simulink model "simulink_scope"  (R2015b)
settings: Solver=VariableStepAuto  StartTime=0.0  StopTime=inf  RelTol=1e-3
undefined symbols (not defined in the file): CR, serial
libraries: instrumentlib x3
settings Model: Creator=adamlang  LastModifiedBy=adamlang

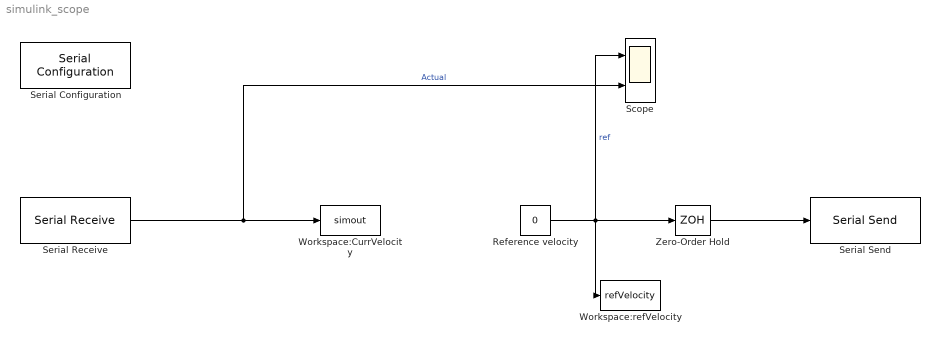
== system simulink_scope ==
  Reference velocity : Constant  Value=0  OutDataTypeStr=single
  Scope : Scope  NumInputPorts=2
  Serial Configuration : instrumentlib/Serial Configuration  Priority=-200000  ComPortMenu=COM75  ComPort=COM75  ObjConstructor=serial('COM75');  BaudRate=115200  DataBits=8  Parity=none  StopBits=1  FlowControl=none  Timeout=10  ByteOrder=LittleEndian
  Serial Receive : instrumentlib/Serial Receive  ComPortMenu=COM75  ComPort=COM75  ObjConstructor=serial('COM75');  Terminator=<none>  DataSize=[1 1]  DataType=single  EnableBlockingMode=on  ActionDataUnavailable=Output last received value  CustomValue=0  SampleTime=0.01
  Serial Send : instrumentlib/Serial Send  ComPortMenu=COM75  ComPort=COM75  ObjConstructor=serial('COM75');  Terminator=CR ('\r')  EnableBlockingMode=on
  Workspace:CurrVelocity : ToWorkspace  VariableName=simout  SaveFormat=Timeseries  SampleTime=-1
  Workspace:refVelocity : ToWorkspace  VariableName=refVelocity  SaveFormat=Timeseries  SampleTime=-1
  Zero-Order Hold : ZeroOrderHold  SampleTime=0.05
  wires:
  Serial Receive/1 -> Scope/2, Workspace:CurrVelocity/1  "Actual"
  Reference velocity/1 -> Workspace:refVelocity/1, Zero-Order Hold/1, Scope/1  "ref"
  Zero-Order Hold/1 -> Serial Send/1
